simulink model "float_sch_TemplateMatchingCentered"  (R2020a)
settings: Solver=VariableStepAuto  StartTime=0  StopTime=10  RelTol=1e-3
values from neighbouring files (symbols this model uses):
  buffer_rec = length(template)    [float_sch_run_TemplateMatchingCentered.m]    (also in float_sch_run_TemplateMatchingContinuous.m)
  delay = round(length(template)/2)    [float_sch_run_TemplateMatchingCentered.m]
  fs = 30000    [float_sch_run_TemplateMatchingCentered.m]    (also in float_sch_run_TemplateMatchingContinuous.m)
  refractory = 10^-3    (= 0.001)    [float_sch_run_TemplateMatchingCentered.m]    (also in float_sch_run_TemplateMatchingContinuous.m)
  score = [3000]    [float_sch_run_TemplateMatchingCentered.m]    (also in float_sch_run_TemplateMatchingContinuous.m = [3600])
  template = double(mean_waveform{1, 2}(:,str2num(ch(3:end))))'    [float_sch_run_TemplateMatchingCentered.m]    (also in float_sch_run_TemplateMatchingContinuous.m = double(mean_waveform{1, 1})')
  th = 70    [float_sch_run_TemplateMatchingCentered.m]
libraries: simulink x3, dspfdesign x2, dspswit3 x1, hdlsllib x1
settings Model: Creator=sbuccelli  LastModifiedBy=diflo

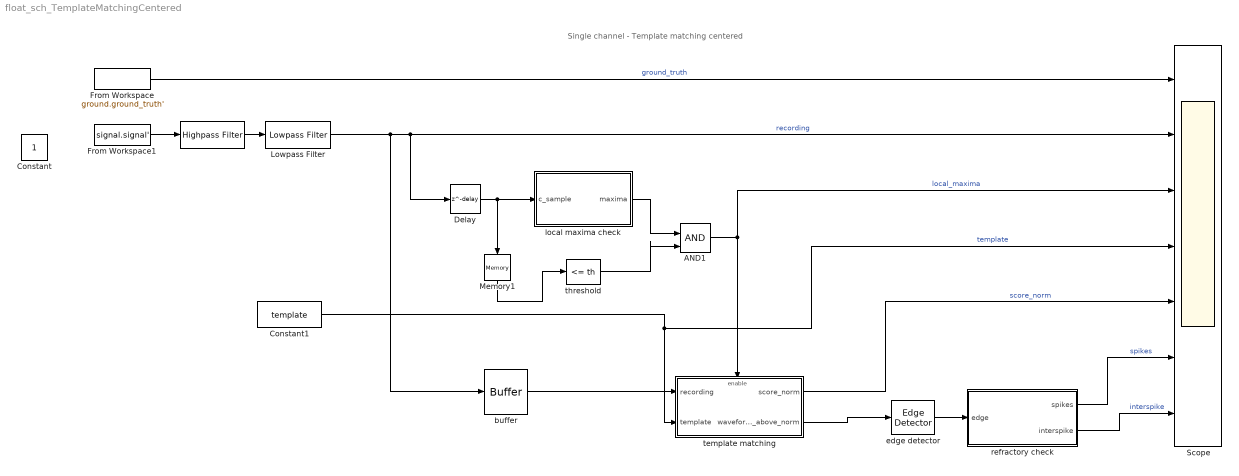
== system float_sch_TemplateMatchingCentered ==
  note: Single channel - Template matching centered
  " " : dspfdesign/Highpass Filter  FilterType=IIR  DesignForMinimumOrder=on  FilterOrder=50  StopbandFrequency=1  PassbandFrequency=300  StopbandAttenuation=80  PassbandRipple=0.1  InheritSampleRate=off  SampleRate=fs  SimulateUsing=Interpreted execution  roundingMode=Floor  coeffsDataTypeStr=fixdt(1,16)
  AND1 : Logic  IconShape=distinctive  AllPortsSameDT=off
  Constant1 : Constant  Value=template
  Delay : Delay  DelayLength=delay  InitialCondition=0
  From Workspace : FromWorkspace  VariableName=ground.ground_truth'  SampleTime=1/fs
  From Workspace1 : FromWorkspace  VariableName=signal.signal'  SampleTime=1/fs
  Lowpass Filter : dspfdesign/Lowpass Filter  FilterType=IIR  DesignForMinimumOrder=on  FilterOrder=3  PassbandFrequency=3500  StopbandFrequency=8500  PassbandRipple=0.1  StopbandAttenuation=80  InheritSampleRate=off  SampleRate=fs  SimulateUsing=Interpreted execution  roundingMode=Floor  coeffsDataTypeStr=fixdt(1,16)
  Memory1 : Memory  InheritSampleTime=on
  Scope : Scope  NumInputPorts=7
  buffer : Buffer  N=buffer_rec  V=buffer_overlap  OutputFrames=off
  edge detector : dspswit3/Edge Detector  InputProcessing=Columns as channels (frame based)
      settings: SourceProductBaseCode=DS
  local maxima check : Subsystem
  refractory check : Subsystem
  template matching : Subsystem
  threshold : simulink/Logic and Bit Operations/Compare To Constant  relop=<=  const=th  OutDataTypeStr=boolean
  Constant : Constant  IOType=siggen
  wires:
  Delay/1 -> Memory1/1, local maxima check/1(c_sample)
  Memory1/1 -> threshold/1
  local maxima check/1(maxima) -> AND1/1
  threshold/1 -> AND1/2
  AND1/1 -> template matching/Enable, Scope/3  "local_maxima"
  edge detector/1 -> refractory check/1("  edge")
  template matching/2(waveform_above_norm) -> edge detector/1
  buffer/1 -> template matching/1(recording)
  Constant1/1 -> Scope/4, template matching/2(template)  "template"
  template matching/1(score_norm) -> Scope/5  "score_norm"
  refractory check/1(" spikes") -> Scope/6  "spikes"
  refractory check/2(interspike) -> Scope/7  "interspike"
  From Workspace/1 -> Scope/1  "ground_truth"
  " "/1 -> Lowpass Filter/1
  From Workspace1/1 -> " "/1
  Lowpass Filter/1 -> buffer/1, Delay/1, Scope/2  "recording"

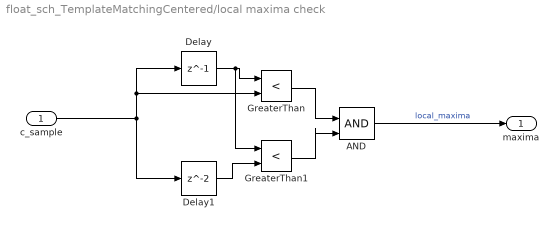
== system float_sch_TemplateMatchingCentered/local maxima check ==
  c_sample : Inport
  AND : Logic  IconShape=distinctive  AllPortsSameDT=off  OutDataTypeStr=boolean
  Delay : Delay  DelayLength=1  SampleTime=1/30000
  Delay1 : Delay  SampleTime=1/30000
  GreaterThan : RelationalOperator  Operator=<  OutDataTypeStr=boolean  RndMeth=Simplest
  GreaterThan1 : RelationalOperator  Operator=<  OutDataTypeStr=boolean  RndMeth=Simplest
  maxima : Outport
  wires:
  Delay/1 -> GreaterThan1/1, GreaterThan/1
  c_sample/1 -> Delay/1, GreaterThan/2, Delay1/1
  GreaterThan/1 -> AND/1
  GreaterThan1/1 -> AND/2
  AND/1 -> maxima/1  "local_maxima"
  Delay1/1 -> GreaterThan1/2

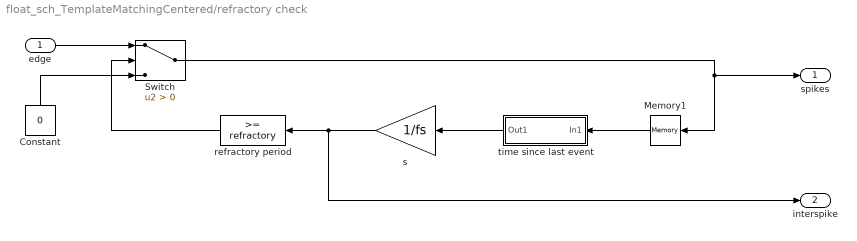
== system float_sch_TemplateMatchingCentered/refractory check ==
  "  edge" : Inport
  Constant : Constant  Value=0
  Memory1 : Memory  InheritSampleTime=on
  Switch : Switch  Criteria=u2 > Threshold
  refractory period : simulink/Logic and Bit Operations/Compare To Constant  relop=>=  const=refractory  OutDataTypeStr=boolean
  s : Gain  Gain=1/fs  ParamDataTypeStr=double
  time since last event : Subsystem
  " spikes" : Outport
  interspike : Outport  Port=2
  wires:
  "  edge"/1 -> Switch/1
  Memory1/1 -> time since last event/1(In1)
  time since last event/1(Out1) -> s/1
  Constant/1 -> Switch/3
  s/1 -> refractory period/1, interspike/1
  Switch/1 -> " spikes"/1, Memory1/1
  refractory period/1 -> Switch/2

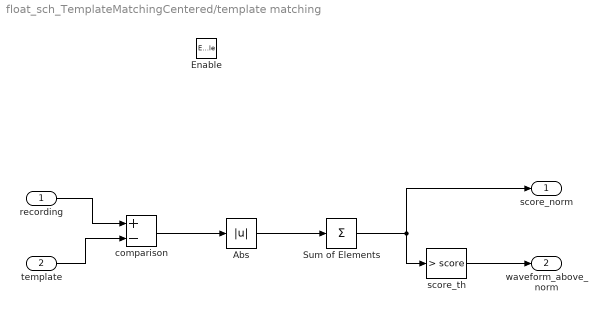
== system float_sch_TemplateMatchingCentered/template matching ==
  recording : Inport
  template : Inport  Port=2
  Enable : EnablePort  StatesWhenEnabling=reset
  Abs : Abs
  Sum of Elements : Sum  Inputs=+
  comparison : Sum  Inputs=+-
  score_th : simulink/Logic and Bit Operations/Compare To Constant  relop=>  const=score  OutDataTypeStr=boolean
  score_norm : Outport  OutputWhenDisabled=reset  InitialOutput=0
  waveform_above_norm : Outport  Port=2
  wires:
  Abs/1 -> Sum of Elements/1
  comparison/1 -> Abs/1
  Sum of Elements/1 -> score_th/1, score_norm/1
  score_th/1 -> waveform_above_norm/1
  recording/1 -> comparison/1
  template/1 -> comparison/2

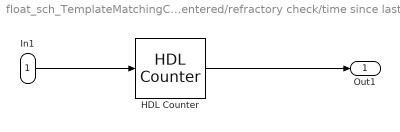
== system float_sch_TemplateMatchingCentered/refractory check/time since last event ==
  In1 : Inport
  HDL Counter : hdlsllib/Sources/HDL Counter  CountType=Free running  CountInit=1  CountStep=1  CountMax=25  CountFromType=Initial value  CountFrom=1  CountResetPort=on  CountLoadPort=off  CountEnbPort=off  CountDirPort=off  CountDataType=Unsigned  CountWordLen=32  CountFracLen=0  CountSampTime=1
  Out1 : Outport
  wires:
  In1/1 -> HDL Counter/1
  HDL Counter/1 -> Out1/1
